simulink model "inLoopSimu_adapt"  (R2024a)
settings: Solver=ode4  StartTime=0.0  StopTime=20000  FixedStep=1E-4  RelTol=1e-3
values from neighbouring files (symbols this model uses):
  estimator =     [ma.mat]    (also in regulation.mat)
  estimator1 =     [ma.mat]
  initial_1 =     [ma.mat]    (also in regulation.mat)
  observer =     [ma.mat]    (also in regulation.mat)
undefined symbols (not defined in the file or in its folder): IAU
libraries: aerolibtransform2 x1
settings Model: Creator=b_ant  LastModifiedBy=b_ant

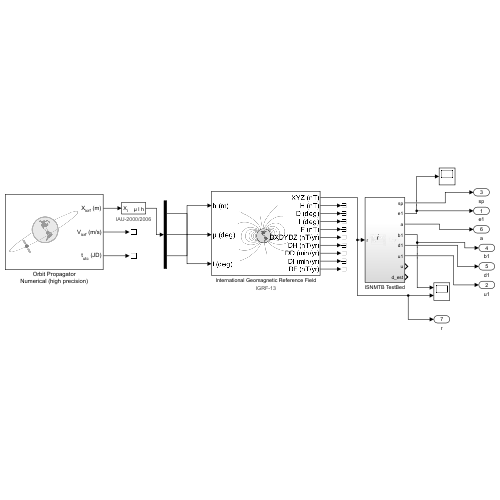
[thumbnail: Simulink's stored preview of the top-level diagram]
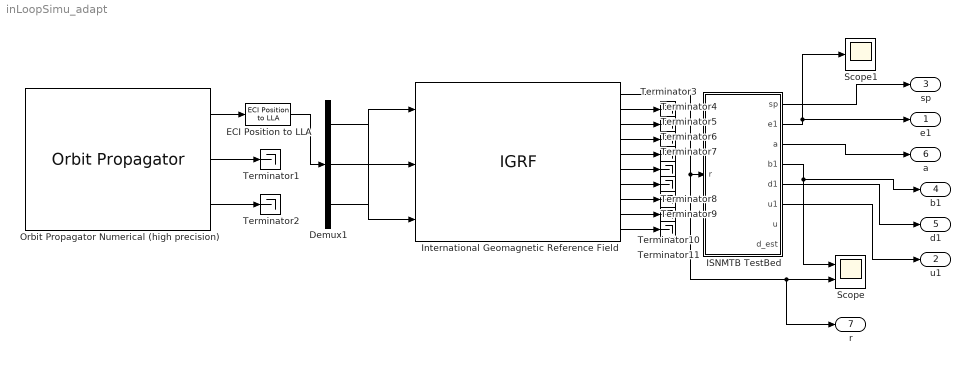
== system inLoopSimu_adapt ==
  Demux1 : Demux  Outputs=3
  ECI Position to LLA : aerolibtransform2/ECI Position to LLA  red=IAU-2000/2006  year=2020  month=January  day=1  hour=0  min=0  sec=0  deltaT=None  errorflag=Error  extraparamflag=off  eunits=Metric (MKS)  earthmodel=WGS84  flat=1/298.257223563  eqradius=6378137
      settings: AttributesFormatString=%<red>
  ISNMTB TestBed : Subsystem
  International Geomagnetic Reference Field : IGRF  time_in=off  month=January  day=1  year=2020
      settings: AttributesFormatString=%<generation>
  Orbit Propagator Numerical (high precision) : OrbitPropagator  accelFrame=Fixed-frame  outportFrame=Fixed-frame  semiMajorAxis=orbit.semiMajorAxis  eccentricity=orbit.eccentricity  inclination=orbit.inclination  raan=orbit.rightAscensionOfAscendingNode  argPeriapsis=orbit.argumentOfPeriapsis  trueAnomaly=orbit.trueAnomaly  inertialPosition=[3649700.0 3308200.0 -4676600.0]  inertialVelocity=[-2750.8 6666.4 2573.4]  fixedPosition=[-4142689.0 -2676864.7 -4669861.6]  fixedVelocity=[1452.7 -6720.7 2568.1]  gravityModel=None  customR=3396200  customMu=4.305e13  customJ2=1.0826269e-03  customOmega=4.06125949e-3  outputTransform=on
  Scope : Scope  NumInputPorts=2
  Scope1 : Scope
  Terminator{1..11} (11 alike) : Terminator
  e1 : Outport
  u1 : Outport  Port=2
  sp : Outport  Port=3
  b1 : Outport  Port=4
  d1 : Outport  Port=5
  a : Outport  Port=6
  r : Outport  Port=7
  wires:
  International Geomagnetic Reference Field/2 -> Terminator3/1
  International Geomagnetic Reference Field/5 -> Terminator6/1
  ECI Position to LLA/1 -> Demux1/1
  Demux1/3 -> International Geomagnetic Reference Field/1
  Orbit Propagator Numerical (high precision)/2 -> Terminator1/1
  Demux1/1 -> International Geomagnetic Reference Field/2
  Orbit Propagator Numerical (high precision)/1 -> ECI Position to LLA/1
  Orbit Propagator Numerical (high precision)/3 -> Terminator2/1
  Demux1/2 -> International Geomagnetic Reference Field/3
  International Geomagnetic Reference Field/3 -> Terminator4/1
  International Geomagnetic Reference Field/9 -> Terminator10/1
  International Geomagnetic Reference Field/6 -> Terminator7/1
  International Geomagnetic Reference Field/4 -> Terminator5/1
  International Geomagnetic Reference Field/10 -> Terminator11/1
  International Geomagnetic Reference Field/7 -> Terminator8/1
  International Geomagnetic Reference Field/8 -> Terminator9/1
  International Geomagnetic Reference Field/1 -> r/1, Scope/2, ISNMTB TestBed/1(r)
  ISNMTB TestBed/1(sp) -> sp/1
  ISNMTB TestBed/2(e1) -> Scope1/1, e1/1
  ISNMTB TestBed/3(a) -> a/1
  ISNMTB TestBed/4(b1) -> Scope/1, b1/1
  ISNMTB TestBed/5(d1) -> d1/1
  ISNMTB TestBed/6(u1) -> u1/1

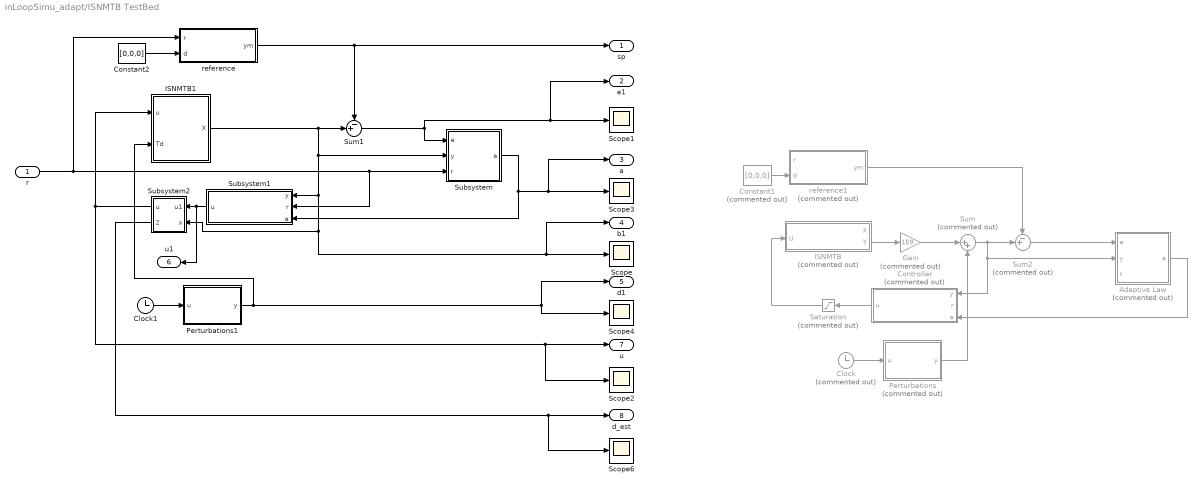
== system inLoopSimu_adapt/ISNMTB TestBed ==
  r : Inport
  Adaptive Law : Subsystem  Commented=on
  Clock : Clock  Commented=on
      settings: Decimation=1000
  Clock1 : Clock
      settings: Decimation=1000
  Constant1 : Constant  Commented=on  Value=[0,0,0]
  Constant2 : Constant  Value=[0,0,0]
  Controller : Subsystem  Commented=on
  Gain : Gain  Commented=on  Gain=1E9
  ISNMTB : Subsystem  Commented=on
  ISNMTB1 : Subsystem
  Perturbations : MATLAB Function  Commented=on  TreatAsAtomicUnit=on
  Perturbations1 : MATLAB Function  TreatAsAtomicUnit=on
  Saturation : Saturate  Commented=on  UpperLimit=[15,7,20]'  LowerLimit=[-15,-7,-25]'
  Scope{,1..4,6} (6 alike) : Scope
  Subsystem : Subsystem
  Subsystem1 : Subsystem
  Subsystem2 : Subsystem
  Sum : Sum  Commented=on  Inputs=|++
  Sum1 : Sum  Inputs=-+|
  Sum2 : Sum  Commented=on  Inputs=-+|
  reference : Subsystem
  reference1 : Subsystem  Commented=on
  sp : Outport
  e1 : Outport  Port=2
  a : Outport  Port=3
  b1 : Outport  Port=4
  d1 : Outport  Port=5
  u1 : Outport  Port=6
  u : Outport  Port=7
  d_est : Outport  Port=8
  wires:
  Sum2/1 -> Adaptive Law/1(e)
  Sum/1 -> Adaptive Law/2(y), Controller/1(y), Sum2/2
  Saturation/1 -> ISNMTB/1(U)
  Adaptive Law/1(a) -> Controller/3(a)
  reference1/1(ym) -> Sum2/1
  Perturbations/1(y) -> Sum/2
  Controller/1(u) -> Saturation/1
  Clock/1 -> Perturbations/1(u)
  Gain/1 -> Sum/1
  ISNMTB/2(Y) -> Gain/1
  Constant1/1 -> reference1/2(d)
  Perturbations1/1(y) -> ISNMTB1/2(Td), d1/1, Scope4/1
  Subsystem2/1(u) -> u/1, Scope2/1, ISNMTB1/1(u)
  Subsystem1/1(u) -> u1/1, Subsystem2/1(u1)
  Constant2/1 -> reference/2(d)
  Subsystem2/2(d_est) -> d_est/1, Scope6/1
  reference/1(ym) -> sp/1, Sum1/1
  Sum1/1 -> Subsystem/1(e), Scope1/1, e1/1
  Subsystem/1(a) -> Subsystem1/3(a), Scope3/1, a/1
  ISNMTB1/1(X) -> Subsystem/2(y), Subsystem2/2(x), Scope/1, b1/1, Subsystem1/1(y), Sum1/2
  Clock1/1 -> Perturbations1/1(u)
  r/1 -> reference/1(r), Subsystem1/2(r), Subsystem/3(r)

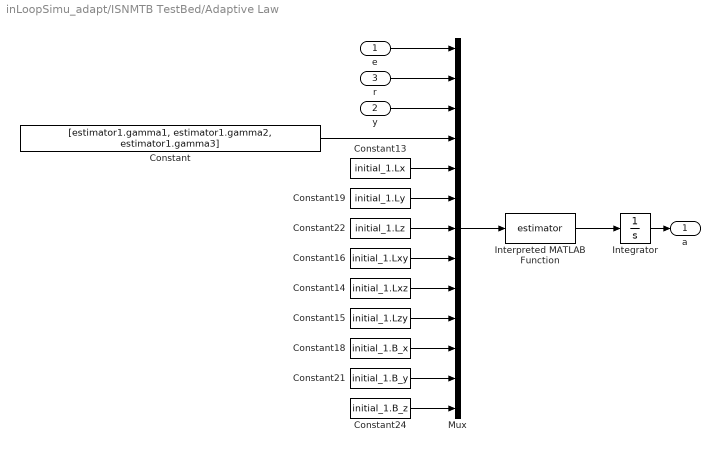
== system inLoopSimu_adapt/ISNMTB TestBed/Adaptive Law ==
  e : Inport
  y : Inport  Port=2
  r : Inport  Port=3
  Constant : Constant  Value=[estimator1.gamma1, estimator1.gamma2, estimator1.gamma3]
  Constant13 : Constant  Value=initial_1.Lx
  Constant14 : Constant  Value=initial_1.Lxz
  Constant15 : Constant  Value=initial_1.Lzy
  Constant16 : Constant  Value=initial_1.Lxy
  Constant18 : Constant  Value=initial_1.B_x
  Constant19 : Constant  Value=initial_1.Ly
  Constant21 : Constant  Value=initial_1.B_y
  Constant22 : Constant  Value=initial_1.Lz
  Constant24 : Constant  Value=initial_1.B_z
  Integrator : Integrator  InitialCondition=[0,0,0,0,0,0]
  Interpreted MATLAB Function : MATLABFcn  MATLABFcn=estimator  OutputDimensions=6
  Mux : Mux  Inputs=13
  a : Outport
  wires:
  Constant21/1 -> Mux/12
  Constant19/1 -> Mux/6
  Constant/1 -> Mux/4
  Constant16/1 -> Mux/8
  Constant18/1 -> Mux/11
  y/1 -> Mux/3
  Constant24/1 -> Mux/13
  Constant13/1 -> Mux/5
  Constant22/1 -> Mux/7
  Interpreted MATLAB Function/1 -> Integrator/1
  r/1 -> Mux/2
  Constant14/1 -> Mux/9
  Constant15/1 -> Mux/10
  Mux/1 -> Interpreted MATLAB Function/1
  e/1 -> Mux/1
  Integrator/1 -> a/1

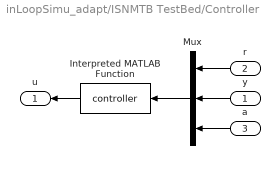
== system inLoopSimu_adapt/ISNMTB TestBed/Controller ==
  y : Inport
  r : Inport  Port=2
  a : Inport  Port=3
  Interpreted MATLAB Function : MATLABFcn  MATLABFcn=controller
  Mux : Mux  Inputs=3
  u : Outport
  wires:
  Mux/1 -> Interpreted MATLAB Function/1
  Interpreted MATLAB Function/1 -> u/1
  a/1 -> Mux/3
  r/1 -> Mux/1
  y/1 -> Mux/2

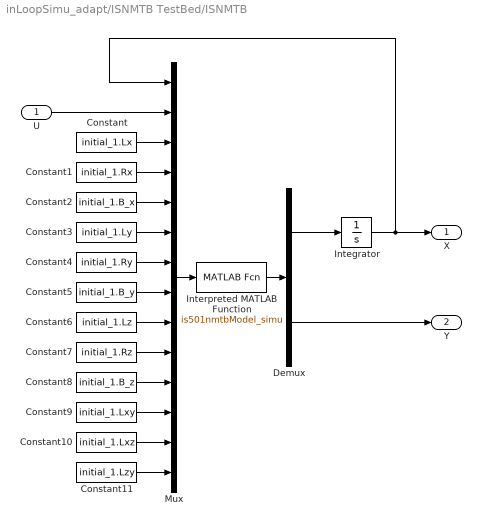
== system inLoopSimu_adapt/ISNMTB TestBed/ISNMTB ==
  U : Inport
  Constant : Constant  Value=initial_1.Lx
  Constant1 : Constant  Value=initial_1.Rx
  Constant10 : Constant  Value=initial_1.Lxz
  Constant11 : Constant  Value=initial_1.Lzy
  Constant2 : Constant  Value=initial_1.B_x
  Constant3 : Constant  Value=initial_1.Ly
  Constant4 : Constant  Value=initial_1.Ry
  Constant5 : Constant  Value=initial_1.B_y
  Constant6 : Constant  Value=initial_1.Lz
  Constant7 : Constant  Value=initial_1.Rz
  Constant8 : Constant  Value=initial_1.B_z
  Constant9 : Constant  Value=initial_1.Lxy
  Demux : Demux  Outputs=2
  Integrator : Integrator  InitialCondition=[0,0,0]
  Interpreted MATLAB Function : MATLABFcn  MATLABFcn=is501nmtbModel_simu  OutputDimensions=6
  Mux : Mux  Inputs=14
  X : Outport
  Y : Outport  Port=2
  wires:
  Constant2/1 -> Mux/5
  Constant/1 -> Mux/3
  Demux/1 -> Integrator/1
  Interpreted MATLAB Function/1 -> Demux/1
  Constant9/1 -> Mux/12
  Constant5/1 -> Mux/8
  Constant3/1 -> Mux/6
  Constant1/1 -> Mux/4
  Integrator/1 -> X/1, Mux/1
  Mux/1 -> Interpreted MATLAB Function/1
  Constant10/1 -> Mux/13
  Constant7/1 -> Mux/10
  Constant11/1 -> Mux/14
  Constant4/1 -> Mux/7
  Constant8/1 -> Mux/11
  Constant6/1 -> Mux/9
  U/1 -> Mux/2
  Demux/2 -> Y/1

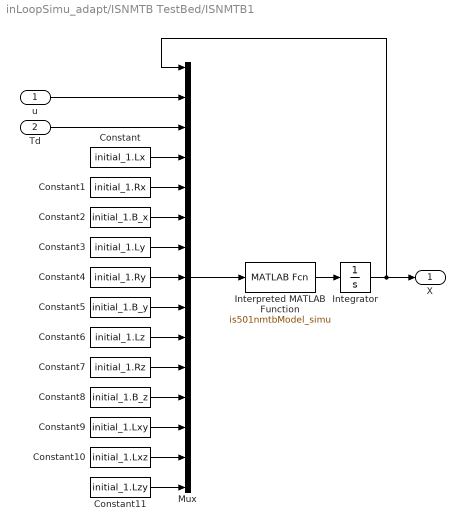
== system inLoopSimu_adapt/ISNMTB TestBed/ISNMTB1 ==
  u : Inport
  Td : Inport  Port=2
  Constant : Constant  Value=initial_1.Lx
  Constant1 : Constant  Value=initial_1.Rx
  Constant10 : Constant  Value=initial_1.Lxz
  Constant11 : Constant  Value=initial_1.Lzy
  Constant2 : Constant  Value=initial_1.B_x
  Constant3 : Constant  Value=initial_1.Ly
  Constant4 : Constant  Value=initial_1.Ry
  Constant5 : Constant  Value=initial_1.B_y
  Constant6 : Constant  Value=initial_1.Lz
  Constant7 : Constant  Value=initial_1.Rz
  Constant8 : Constant  Value=initial_1.B_z
  Constant9 : Constant  Value=initial_1.Lxy
  Integrator : Integrator  InitialCondition=[3.249E4, -2.265E4, 3.655E4]
  Interpreted MATLAB Function : MATLABFcn  MATLABFcn=is501nmtbModel_simu
  Mux : Mux  Inputs=15
  X : Outport
  wires:
  Interpreted MATLAB Function/1 -> Integrator/1
  Integrator/1 -> X/1, Mux/1
  Mux/1 -> Interpreted MATLAB Function/1
  u/1 -> Mux/2
  Td/1 -> Mux/3
  Constant/1 -> Mux/4
  Constant1/1 -> Mux/5
  Constant2/1 -> Mux/6
  Constant3/1 -> Mux/7
  Constant4/1 -> Mux/8
  Constant5/1 -> Mux/9
  Constant6/1 -> Mux/10
  Constant7/1 -> Mux/11
  Constant8/1 -> Mux/12
  Constant9/1 -> Mux/13
  Constant10/1 -> Mux/14
  Constant11/1 -> Mux/15

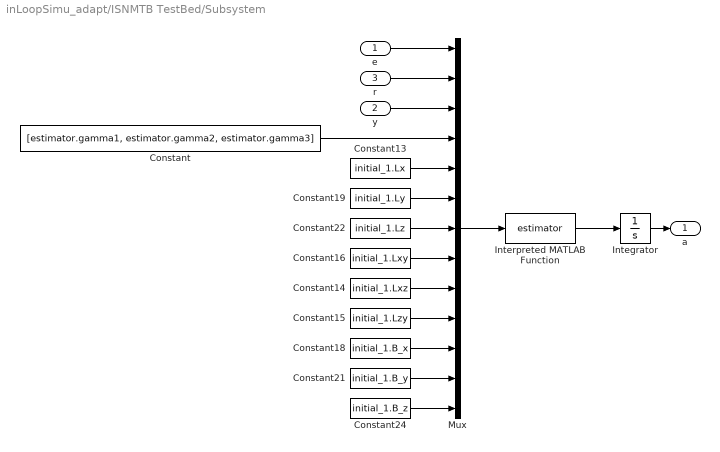
== system inLoopSimu_adapt/ISNMTB TestBed/Subsystem ==
  e : Inport
  y : Inport  Port=2
  r : Inport  Port=3
  Constant : Constant  Value=[estimator.gamma1, estimator.gamma2, estimator.gamma3]
  Constant13 : Constant  Value=initial_1.Lx
  Constant14 : Constant  Value=initial_1.Lxz
  Constant15 : Constant  Value=initial_1.Lzy
  Constant16 : Constant  Value=initial_1.Lxy
  Constant18 : Constant  Value=initial_1.B_x
  Constant19 : Constant  Value=initial_1.Ly
  Constant21 : Constant  Value=initial_1.B_y
  Constant22 : Constant  Value=initial_1.Lz
  Constant24 : Constant  Value=initial_1.B_z
  Integrator : Integrator  InitialCondition=[0,0,0,0,0,0]
  Interpreted MATLAB Function : MATLABFcn  MATLABFcn=estimator  OutputDimensions=6
  Mux : Mux  Inputs=13
  a : Outport
  wires:
  Constant21/1 -> Mux/12
  Constant19/1 -> Mux/6
  Constant/1 -> Mux/4
  Constant16/1 -> Mux/8
  Constant18/1 -> Mux/11
  y/1 -> Mux/3
  Constant24/1 -> Mux/13
  Constant13/1 -> Mux/5
  Constant22/1 -> Mux/7
  Interpreted MATLAB Function/1 -> Integrator/1
  r/1 -> Mux/2
  Constant14/1 -> Mux/9
  Constant15/1 -> Mux/10
  Mux/1 -> Interpreted MATLAB Function/1
  e/1 -> Mux/1
  Integrator/1 -> a/1

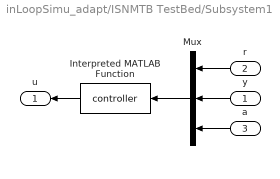
== system inLoopSimu_adapt/ISNMTB TestBed/Subsystem1 ==
  y : Inport
  r : Inport  Port=2
  a : Inport  Port=3
  Interpreted MATLAB Function : MATLABFcn  MATLABFcn=controller
  Mux : Mux  Inputs=3
  u : Outport
  wires:
  Mux/1 -> Interpreted MATLAB Function/1
  Interpreted MATLAB Function/1 -> u/1
  a/1 -> Mux/3
  r/1 -> Mux/1
  y/1 -> Mux/2

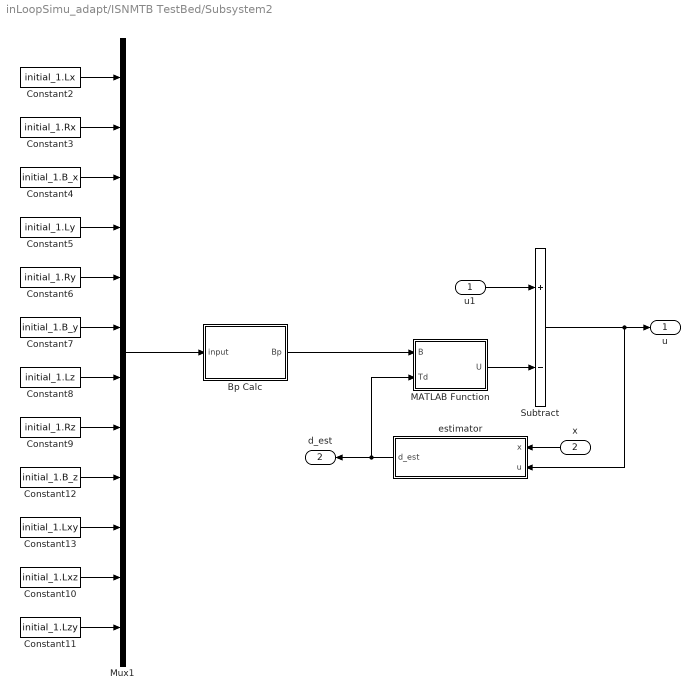
== system inLoopSimu_adapt/ISNMTB TestBed/Subsystem2 ==
  u1 : Inport
  x : Inport  Port=2
  Bp Calc : MATLAB Function  TreatAsAtomicUnit=on
  Constant10 : Constant  Value=initial_1.Lxz
  Constant11 : Constant  Value=initial_1.Lzy
  Constant12 : Constant  Value=initial_1.B_z
  Constant13 : Constant  Value=initial_1.Lxy
  Constant2 : Constant  Value=initial_1.Lx
  Constant3 : Constant  Value=initial_1.Rx
  Constant4 : Constant  Value=initial_1.B_x
  Constant5 : Constant  Value=initial_1.Ly
  Constant6 : Constant  Value=initial_1.Ry
  Constant7 : Constant  Value=initial_1.B_y
  Constant8 : Constant  Value=initial_1.Lz
  Constant9 : Constant  Value=initial_1.Rz
  MATLAB Function : MATLAB Function  TreatAsAtomicUnit=on
  Mux1 : Mux  Inputs=12
  Subtract : Sum  Inputs=+-
  estimator : Subsystem
  u : Outport
  d_est : Outport  Port=2
  wires:
  Constant6/1 -> Mux1/5
  Constant4/1 -> Mux1/3
  estimator/1(d_est) -> d_est/1, MATLAB Function/2(Td)
  Constant2/1 -> Mux1/1
  Constant10/1 -> Mux1/11
  Constant13/1 -> Mux1/10
  Constant5/1 -> Mux1/4
  Constant12/1 -> Mux1/9
  Constant3/1 -> Mux1/2
  Constant9/1 -> Mux1/8
  Mux1/1 -> Bp Calc/1(input)
  Constant7/1 -> Mux1/6
  Constant8/1 -> Mux1/7
  Constant11/1 -> Mux1/12
  Bp Calc/1(Bp) -> MATLAB Function/1(B)
  x/1 -> estimator/1(x)
  Subtract/1 -> estimator/2(u), u/1
  MATLAB Function/1(U) -> Subtract/2
  u1/1 -> Subtract/1

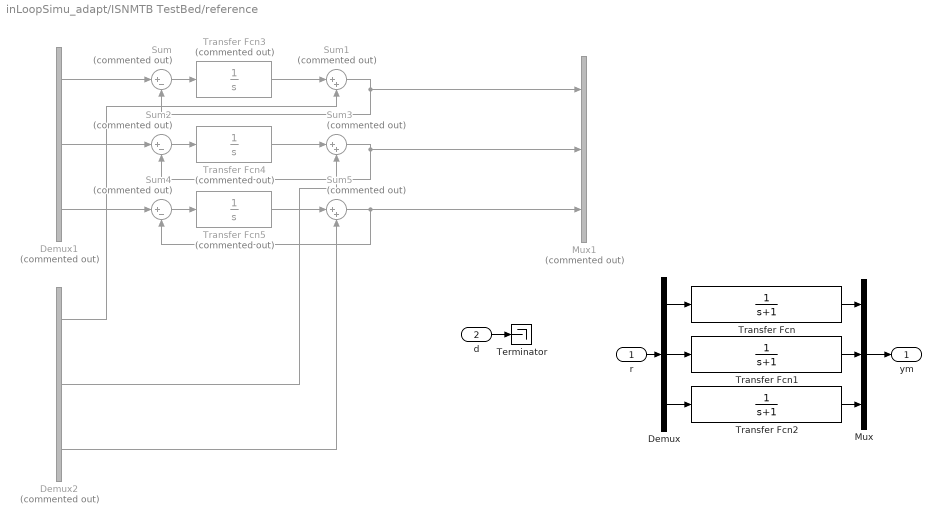
== system inLoopSimu_adapt/ISNMTB TestBed/reference ==
  r : Inport
  d : Inport  Port=2
  Demux : Demux  Outputs=3
  Demux1 : Demux  Commented=on  Outputs=3
  Demux2 : Demux  Commented=on  Outputs=3
  Mux : Mux  Inputs=3
  Mux1 : Mux  Commented=on  Inputs=3
  Sum : Sum  Commented=on  Inputs=|+-
  Sum1 : Sum  Commented=on  Inputs=|++
  Sum2 : Sum  Commented=on  Inputs=|+-
  Sum3 : Sum  Commented=on  Inputs=|++
  Sum4 : Sum  Commented=on  Inputs=|+-
  Sum5 : Sum  Commented=on  Inputs=|++
  Terminator : Terminator
  Transfer Fcn : TransferFcn  Numerator=1  Denominator=[1 1]
  Transfer Fcn1 : TransferFcn  Numerator=1  Denominator=[1 1]
  Transfer Fcn2 : TransferFcn  Numerator=1  Denominator=[1 1]
  Transfer Fcn3 : TransferFcn  Commented=on  Numerator=1  Denominator=[1 0]
  Transfer Fcn4 : TransferFcn  Commented=on  Numerator=1  Denominator=[1 0]
  Transfer Fcn5 : TransferFcn  Commented=on  Numerator=1  Denominator=[1 0]
  ym : Outport
  wires:
  Demux/2 -> Transfer Fcn1/1
  Transfer Fcn/1 -> Mux/1
  Demux/1 -> Transfer Fcn/1
  Demux/3 -> Transfer Fcn2/1
  Transfer Fcn1/1 -> Mux/2
  Transfer Fcn2/1 -> Mux/3
  Sum5/1 -> Sum4/2, Mux1/3
  Sum3/1 -> Sum2/2, Mux1/2
  Demux1/1 -> Sum/1
  Sum/1 -> Transfer Fcn3/1
  Transfer Fcn3/1 -> Sum1/1
  Sum1/1 -> Sum/2, Mux1/1
  Sum2/1 -> Transfer Fcn4/1
  Transfer Fcn4/1 -> Sum3/1
  Sum4/1 -> Transfer Fcn5/1
  Transfer Fcn5/1 -> Sum5/1
  Demux1/2 -> Sum2/1
  Demux1/3 -> Sum4/1
  Demux2/1 -> Sum1/2
  Demux2/2 -> Sum3/2
  Demux2/3 -> Sum5/2
  r/1 -> Demux/1
  Mux/1 -> ym/1
  d/1 -> Terminator/1

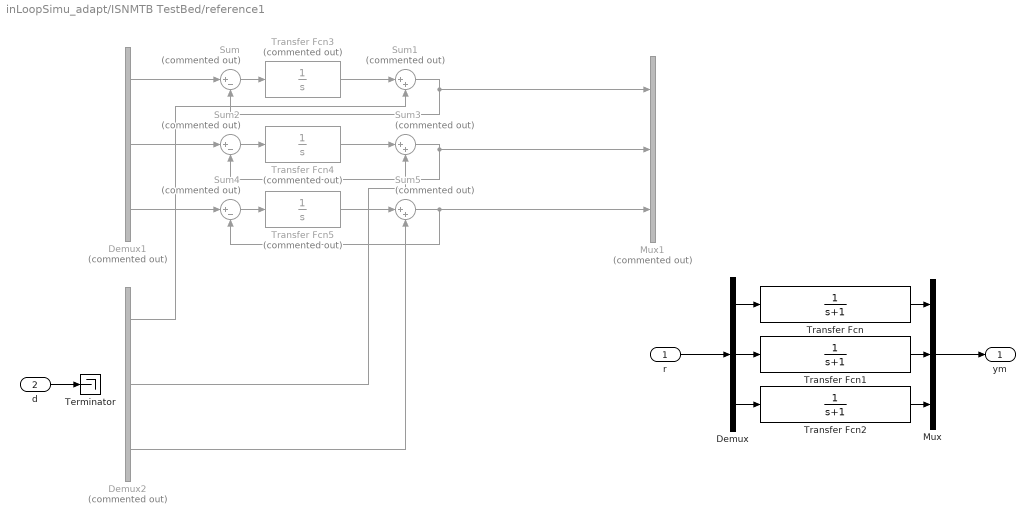
== system inLoopSimu_adapt/ISNMTB TestBed/reference1 ==
  r : Inport
  d : Inport  Port=2
  Demux : Demux  Outputs=3
  Demux1 : Demux  Commented=on  Outputs=3
  Demux2 : Demux  Commented=on  Outputs=3
  Mux : Mux  Inputs=3
  Mux1 : Mux  Commented=on  Inputs=3
  Sum : Sum  Commented=on  Inputs=|+-
  Sum1 : Sum  Commented=on  Inputs=|++
  Sum2 : Sum  Commented=on  Inputs=|+-
  Sum3 : Sum  Commented=on  Inputs=|++
  Sum4 : Sum  Commented=on  Inputs=|+-
  Sum5 : Sum  Commented=on  Inputs=|++
  Terminator : Terminator
  Transfer Fcn : TransferFcn  Numerator=1  Denominator=[1 1]
  Transfer Fcn1 : TransferFcn  Numerator=1  Denominator=[1 1]
  Transfer Fcn2 : TransferFcn  Numerator=1  Denominator=[1 1]
  Transfer Fcn3 : TransferFcn  Commented=on  Numerator=1  Denominator=[1 0]
  Transfer Fcn4 : TransferFcn  Commented=on  Numerator=1  Denominator=[1 0]
  Transfer Fcn5 : TransferFcn  Commented=on  Numerator=1  Denominator=[1 0]
  ym : Outport
  wires:
  Demux/2 -> Transfer Fcn1/1
  Transfer Fcn/1 -> Mux/1
  Demux/1 -> Transfer Fcn/1
  Demux/3 -> Transfer Fcn2/1
  Transfer Fcn1/1 -> Mux/2
  Transfer Fcn2/1 -> Mux/3
  Sum5/1 -> Sum4/2, Mux1/3
  Sum3/1 -> Sum2/2, Mux1/2
  Demux1/1 -> Sum/1
  Sum/1 -> Transfer Fcn3/1
  Transfer Fcn3/1 -> Sum1/1
  Sum1/1 -> Sum/2, Mux1/1
  Sum2/1 -> Transfer Fcn4/1
  Transfer Fcn4/1 -> Sum3/1
  Sum4/1 -> Transfer Fcn5/1
  Transfer Fcn5/1 -> Sum5/1
  Demux1/2 -> Sum2/1
  Demux1/3 -> Sum4/1
  Demux2/1 -> Sum1/2
  Demux2/2 -> Sum3/2
  Demux2/3 -> Sum5/2
  r/1 -> Demux/1
  Mux/1 -> ym/1
  d/1 -> Terminator/1

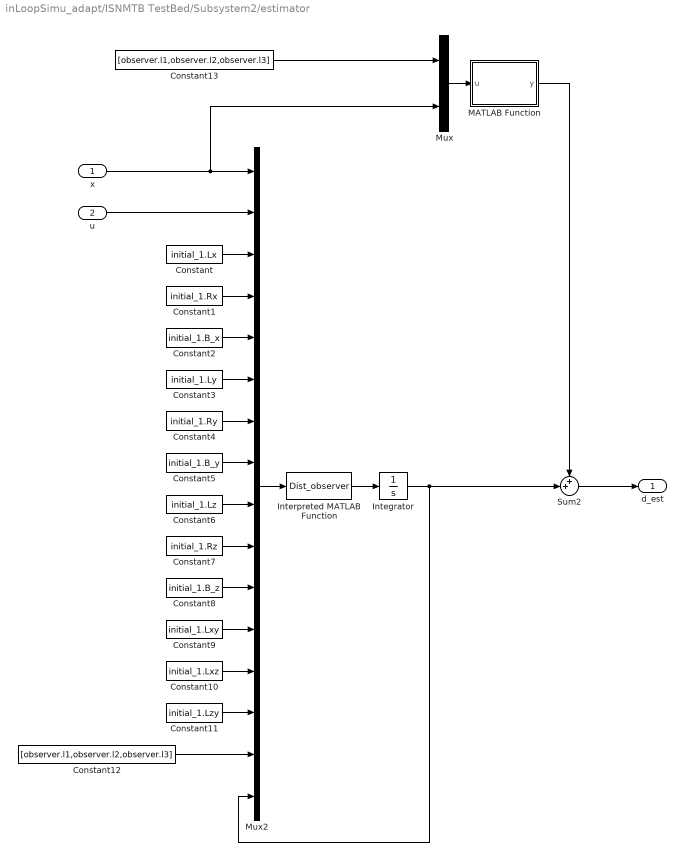
== system inLoopSimu_adapt/ISNMTB TestBed/Subsystem2/estimator ==
  x : Inport
  u : Inport  Port=2
  Constant : Constant  Value=initial_1.Lx
  Constant1 : Constant  Value=initial_1.Rx
  Constant10 : Constant  Value=initial_1.Lxz
  Constant11 : Constant  Value=initial_1.Lzy
  Constant12 : Constant  Value=[observer.l1,observer.l2,observer.l3]
  Constant13 : Constant  Value=[observer.l1,observer.l2,observer.l3]
  Constant2 : Constant  Value=initial_1.B_x
  Constant3 : Constant  Value=initial_1.Ly
  Constant4 : Constant  Value=initial_1.Ry
  Constant5 : Constant  Value=initial_1.B_y
  Constant6 : Constant  Value=initial_1.Lz
  Constant7 : Constant  Value=initial_1.Rz
  Constant8 : Constant  Value=initial_1.B_z
  Constant9 : Constant  Value=initial_1.Lxy
  Integrator : Integrator  InitialCondition=[0,0,0]
  Interpreted MATLAB Function : MATLABFcn  MATLABFcn=Dist_observer
  MATLAB Function : MATLAB Function  TreatAsAtomicUnit=on
  Mux : Mux  Inputs=2
  Mux2 : Mux  Inputs=16
  Sum2 : Sum  Inputs=++|
  d_est : Outport
  wires:
  Constant6/1 -> Mux2/9
  MATLAB Function/1(y) -> Sum2/1
  Constant10/1 -> Mux2/13
  Integrator/1 -> Sum2/2, Mux2/16
  Interpreted MATLAB Function/1 -> Integrator/1
  Constant2/1 -> Mux2/5
  Constant4/1 -> Mux2/7
  Constant7/1 -> Mux2/10
  Mux2/1 -> Interpreted MATLAB Function/1
  Constant11/1 -> Mux2/14
  Constant8/1 -> Mux2/11
  Constant1/1 -> Mux2/4
  Constant3/1 -> Mux2/6
  Constant/1 -> Mux2/3
  Constant9/1 -> Mux2/12
  Constant5/1 -> Mux2/8
  Constant12/1 -> Mux2/15
  u/1 -> Mux2/2
  Sum2/1 -> d_est/1
  Constant13/1 -> Mux/1
  Mux/1 -> MATLAB Function/1(u)
  x/1 -> Mux/2, Mux2/1

== matlab function inLoopSimu_adapt/ISNMTB TestBed/Perturbations1 ==
  data: u input; y output
function y = fcn(u)
y= [2.522*sin(2*pi*4.788E-3*u)+3.249E04;
   -5.174*sin(2*pi*7.481E-3*u)-2.265E04;
    3.359*sin(2*pi*8.378E-3*u)+3.655E04];
end

== matlab function inLoopSimu_adapt/ISNMTB TestBed/Subsystem2/estimator/MATLAB Function ==
  data: u input; y output
function y = fcn(u)
l = diag([u(1),u(2),u(3)]);
x = [u(4);u(5);u(6)];

y = l*x;
end

== matlab function inLoopSimu_adapt/ISNMTB TestBed/Subsystem2/Bp Calc ==
  data: input input; Bp output
function Bp = fcn(input)
    Lxx =  input(1);
    Rx  =  input(2);
    B_1 =  input(3);
    Lyy =  input(4);
    Ry  =  input(5);
    B_2 =  input(6);
    Lzz =  input(7);
    Rz  =  input(8);
    B_3 =  input(9);
    Lxy =  input(10);
    Lxz =  input(11);
    Lzy =  input(12);

    %%%Parameter reading
    L1 =[Lxx, (B_1/B_2)*Lxy, (B_1/B_3)*Lxz;
        (B_2/B_1)*Lxy, Lyy, (B_2/B_3)*Lzy;
        (B_3/B_1)*Lxz, (B_3/B_2)*Lzy, Lzz];
    L = [Lxx, Lxy, Lxz;
         Lxy, Lyy, Lzy;
         Lxz, Lzy, Lzz];
    R = diag([Rx,Ry,Rz]);
    B = diag([B_1,B_2,B_3]);
    
    %%% Model matrix
    %Ap = -inv(L1)*R;
    Bp =  B*inv(L)*1E9;
    %Bp = Bp';
    %Bp_out = Bp(:);
end

== matlab function inLoopSimu_adapt/ISNMTB TestBed/Subsystem2/MATLAB Function ==
  data: B input; U output; Td input
function U = fcn(B,Td)
 U = inv(B)*Td;
end

== matlab function inLoopSimu_adapt/ISNMTB TestBed/Perturbations ==
  data: u input; y output
function y = fcn(u)
y= [2.522*sin(2*pi*4.788E-3*u)+3.249E04;
   -5.174*sin(2*pi*7.481E-3*u)-2.265E04;
    3.359*sin(2*pi*8.378E-3*u)+3.655E04];
end
